simulink model "lipetz"  (R2018b)
settings: Solver=VariableStepAuto  StartTime=0.0  StopTime=20  RelTol=1e-3
libraries: discretizing x4
settings Model: Creator=vsharma98  LastModifiedBy=vsharma98

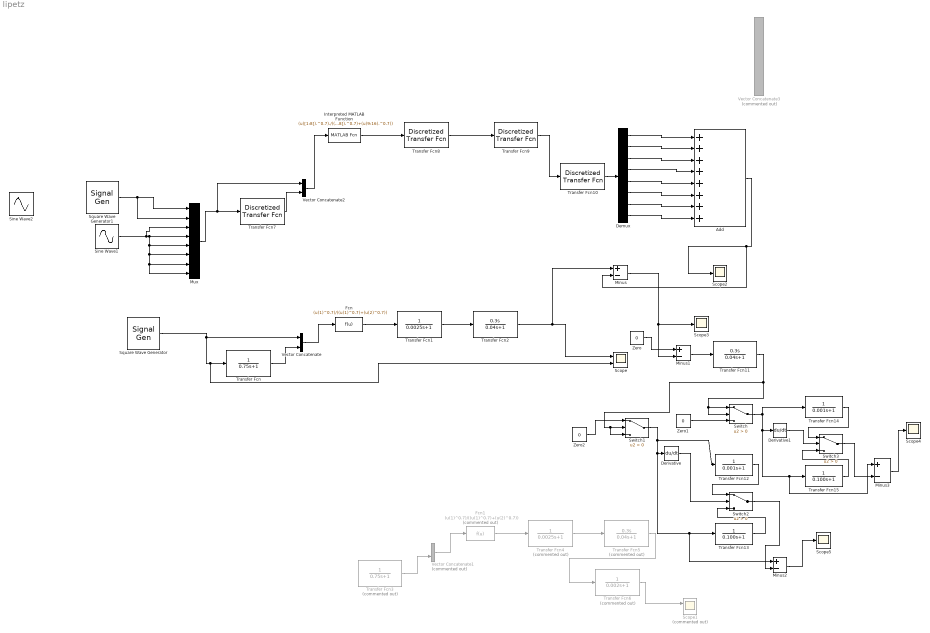
== system lipetz ==
  Add : Sum  Inputs=++++++++
  Demux : Demux  Outputs=8
  Derivative : Derivative
  Derivative1 : Derivative
  Fcn : Fcn  Expr=(u(1)^0.7)/((u(1)^0.7)+(u(2)^0.7))
  Fcn1 : Fcn  Commented=on  Expr=(u(1)^0.7)/((u(1)^0.7)+(u(2)^0.7))
  Interpreted MATLAB Function : MATLABFcn  MATLABFcn=(u([1:8]).^0.7)./((u([1:8]).^0.7)+(u(9:16).^0.7))  Output1D=off
  Minus{,1..3} (4 alike) : Sum  Inputs=+-
  Mux : Mux  Inputs=8
  Scope : Scope  NumInputPorts=2
  Scope1 : Scope  Commented=on  NumInputPorts=2
  Scope{2..5} (4 alike) : Scope
  Sine Wave1 : Sin  Bias=1  Frequency=1*2*pi  SampleTime=0
  Sine Wave2 : Sin  Amplitude=2  Bias=1  Frequency=7.1*2*pi  SampleTime=0
  Square Wave Generator : SignalGenerator  WaveForm=square  Frequency=1*2*pi  Units=rad/sec
  Square Wave Generator1 : SignalGenerator  WaveForm=square  Amplitude=2  Frequency=7.1*2*pi  Units=rad/sec
  Switch{,1..3} (4 alike) : Switch  Criteria=u2 > Threshold
  Transfer Fcn : TransferFcn  Denominator=[0.75 1]
  Transfer Fcn1 : TransferFcn  Denominator=[0.0025 1]
  Transfer Fcn10 : discretizing/Discretized Transfer Fcn  Numerator=[1]  Denominator=[0.002 1]  AbsTol=auto  SampleTime=0.01  method=zoh  Wc=1
  Transfer Fcn11 : TransferFcn  Numerator=[0.3 0]  Denominator=[0.04 1]
  Transfer Fcn12 : TransferFcn  Denominator=[0.001 1]
  Transfer Fcn13 : TransferFcn  Denominator=[0.100 1]
  Transfer Fcn14 : TransferFcn  Denominator=[0.001 1]
  Transfer Fcn15 : TransferFcn  Denominator=[0.100 1]
  Transfer Fcn2 : TransferFcn  Numerator=[0.3 0]  Denominator=[0.04 1]
  Transfer Fcn3 : TransferFcn  Commented=on  Denominator=[0.75 1]
  Transfer Fcn4 : TransferFcn  Commented=on  Denominator=[0.0025 1]
  Transfer Fcn5 : TransferFcn  Commented=on  Numerator=[0.3 0]  Denominator=[0.04 1]
  Transfer Fcn6 : TransferFcn  Commented=on  Denominator=[0.002 1]
  Transfer Fcn7 : discretizing/Discretized Transfer Fcn  Numerator=[1]  Denominator=[0.75 1]  AbsTol=auto  SampleTime=0.01  method=zoh  Wc=1
  Transfer Fcn8 : discretizing/Discretized Transfer Fcn  Numerator=[1]  Denominator=[0.0025 1]  AbsTol=auto  SampleTime=0.01  method=zoh  Wc=1
  Transfer Fcn9 : discretizing/Discretized Transfer Fcn  Numerator=[0.3 0]  Denominator=[0.04 1]  AbsTol=auto  SampleTime=0.01  method=zoh  Wc=1
  Vector Concatenate : Concatenate
  Vector Concatenate1 : Concatenate  Commented=on
  Vector Concatenate2 : Concatenate
  Vector Concatenate3 : Concatenate  Commented=on  NumInputs=8
  Zero : Constant  Value=0  OutDataTypeStr=Inherit: Inherit via back propagation
  Zero1 : Constant  Value=0  OutDataTypeStr=Inherit: Inherit via back propagation
  Zero2 : Constant  Value=0  OutDataTypeStr=Inherit: Inherit via back propagation
  wires:
  Square Wave Generator/1 -> Vector Concatenate/1, Scope/2, Transfer Fcn/1
  Transfer Fcn/1 -> Vector Concatenate/2
  Vector Concatenate/1 -> Fcn/1
  Fcn/1 -> Transfer Fcn1/1
  Transfer Fcn1/1 -> Transfer Fcn2/1
  Transfer Fcn2/1 -> Minus/1, Scope/1
  Transfer Fcn4/1 -> Transfer Fcn5/1
  Vector Concatenate1/1 -> Fcn1/1
  Transfer Fcn3/1 -> Vector Concatenate1/2
  Transfer Fcn5/1 -> Transfer Fcn6/1
  ? -> Vector Concatenate1/1, Scope1/2, Transfer Fcn3/1
  Fcn1/1 -> Transfer Fcn4/1
  Transfer Fcn6/1 -> Scope1/1
  Sine Wave1/1 -> Mux/3, Mux/8, Mux/7, Mux/6, Mux/5, Mux/4
  Mux/1 -> Vector Concatenate2/1, Transfer Fcn7/1
  Demux/3 -> Add/3
  Demux/2 -> Add/2
  Demux/1 -> Add/1
  Transfer Fcn7/1 -> Vector Concatenate2/2
  Vector Concatenate2/1 -> Interpreted MATLAB Function/1
  Demux/4 -> Add/4
  Demux/5 -> Add/5
  Demux/6 -> Add/6
  Demux/7 -> Add/7
  Demux/8 -> Add/8
  Interpreted MATLAB Function/1 -> Transfer Fcn8/1
  Transfer Fcn8/1 -> Transfer Fcn9/1
  Transfer Fcn9/1 -> Transfer Fcn10/1
  Transfer Fcn10/1 -> Demux/1
  Add/1 -> Minus/2, Scope2/1
  Minus/1 -> Minus1/2, Scope3/1
  Zero/1 -> Minus1/1
  Minus1/1 -> Transfer Fcn11/1
  Zero1/1 -> Switch/3
  Switch/1 -> Minus3/1, Transfer Fcn15/1, Derivative1/1, Transfer Fcn14/1
  Transfer Fcn11/1 -> Switch1/3, Switch1/2, Switch/1, Switch/2
  Switch1/1 -> Minus2/1, Transfer Fcn13/1, Derivative/1, Transfer Fcn12/1
  Zero2/1 -> Switch1/1
  Derivative/1 -> Switch2/2
  Derivative1/1 -> Switch3/2
  Transfer Fcn12/1 -> Switch2/1
  Transfer Fcn13/1 -> Switch2/3
  Switch2/1 -> Minus2/2
  Transfer Fcn15/1 -> Switch3/3
  Transfer Fcn14/1 -> Switch3/1
  Switch3/1 -> Minus3/2
  Minus2/1 -> Scope5/1
  Minus3/1 -> Scope4/1
  Square Wave Generator1/1 -> Mux/2, Mux/1
